simulink model "gm_Test_DOA"  (R2020b)
settings: Solver=ode4  StartTime=0.0  StopTime=0.16  RelTol=1e-3
undefined symbols (not defined in the file or in its folder): f_range, FFT_LENGTH, InvMp, Sampling_rate
libraries: dsphdlmathfun x4, dsphdlxfrm x4, hdlsllib x1
(part 1 of 2)
settings Model: Creator=tigro  LastModifiedBy=franc
settings OptimizationCC: BlockReduction=off  ConditionallyExecuteInputs=off  DefaultParameterBehavior=Inlined  OptimizeBlockIOStorage=off  EnhancedBackFolding=on  PassReuseOutputArgsAs=Individual arguments  OptimizeBlockOrder=speed  DifferentSizesBufferReuse=on  EfficientTunableParamExpr=on
settings DebuggingCC: AlgebraicLoopMsg=error  InheritedTsInSrcMsg=none  ParameterOverflowMsg=none  ParameterTunabilityLossMsg=error  AllowAutomaticUnitConversions=off
settings HardwareCC: ProdBitPerPointer=32  ProdBitPerSizeT=32  ProdBitPerPtrDiffT=32  ProdLargestAtomicFloat=None  ProdIntDivRoundTo=Undefined  ProdEndianess=Unspecified  ProdWordSize=32  ProdHWDeviceType=ASIC/FPGA->ASIC/FPGA  TargetBitPerPointer=64  TargetBitPerSizeT=64  TargetBitPerPtrDiffT=64  TargetLongLongMode=on  TargetIntDivRoundTo=Zero  TargetEndianess=LittleEndian  TargetWordSize=64  TargetHWDeviceType=Generic->Custom  ProdEqTarget=off
settings SFSimCC: MATLABDynamicMemAlloc=off
settings RTWCC: Description=SystemVerilog DPI Component Generator  SystemTargetFile=systemverilog_dpi_ert.tlc  TemplateMakefile=systemverilog_dpi_ert_default_tmf
settings CodeAppCC: ForceParamTrailComments=on  IgnoreCustomStorageClasses=off  MaxIdLength=256  OperatorAnnotations=on  SimulinkDataObjDesc=on  SFDataObjDesc=on  InsertBlockDesc=on
settings DPIERTTargetCC: TargetFcnLib=ansi_tfl_table_tmw.mat  GenFloatMathFcnCalls=NOT IN USE  TargetLangStandard=C89/C90 (ANSI)  CodeReplacementLibrary=None  UtilityFuncGeneration=Auto  MultiwordTypeDef=System defined  MultiwordLength=2048  DynamicStringBufferSize=256  GenerateFullHeader=on  InferredTypesCompatibility=off  GenerateSampleERTMain=off  GenerateTestInterfaces=off  ModelReferenceCompliant=on  ParMdlRefBuildCompliant=on  CompOptLevelCompliant=off  ConcurrentExecutionCompliant=off  IncludeMdlTerminateFcn=on  CombineOutputUpdateFcns=off  CombineSignalStateStructs=on  GroupInternalDataByFunction=off  SuppressErrorStatus=off  IncludeFileDelimiter=Auto  ERTCustomFileBanners=on  SupportAbsoluteTime=on  LogVarNameModifier=rt_  MatFileLogging=off  CodeInterfacePackaging=Reusable function  PurelyIntegerCode=off  SupportNonFinite=on  SupportComplex=on  SupportContinuousTime=on  SupportNonInlinedSFcns=on  RemoveDisableFunc=off  RemoveResetFunc=on  SupportVariableSizeSignals=off  ParenthesesLevel=Nominal  CastingMode=Nominal  MATLABClassNameForMDSCustomization=Simulink.SoftwareTarget.TargetSpecificTriggerConfigurationBase  ModelStepFunctionPrototypeControlCompliant=on  CPPClassGenCompliant=off  AutosarCompliant=off  MDXCompliant=off  GRTInterface=off  GenerateAllocFcn=on  UseToolchainInfoCompliant=on  GenerateSharedConstants=on  CoderGroups=[]  AccessMethods=[]  LookupTableObjectStructAxisOrder=1,2,3,4,...  LUTObjectStructOrderExplicitValues=Size,Breakpoints,Table  LUTObjectStructOrderEvenSpacing=Size,Breakpoints,Table  ArrayLayout=Column-major  UnsupportedSFcnMsg=error  ERTHeaderFileRootName=$R$E  ERTSourceFileRootName=$R$E  ERTDataFileRootName=$R_data  GenerateASAP2=off  DSAsUniqueAccess=off  ExtMode=off  ExtModeTransport=0  ExtModeStaticAlloc=off  ExtModeStaticAllocSize=1000000  ExtModeTesting=off  ExtModeMexFile=ext_comm  ExtModeIntrfLevel=Level1  InlinedParameterPlacement=NonHierarchical  TargetOS=BareBoardExample  MultiInstanceErrorCode=Error  RootIOFormat=Part of model data structure  RTWCAPISignals=on  RTWCAPIParams=off  RTWCAPIStates=off  RTWCAPIRootIO=off  ERTSrcFileBannerTemplate=ert_code_template.cgt  ERTHdrFileBannerTemplate=ert_code_template.cgt  ERTDataSrcFileTemplate=ert_code_template.cgt  ERTDataHdrFileTemplate=ert_code_template.cgt  ERTCustomFileTemplate=example_file_process.tlc  EnableDataOwnership=off  SignalDisplayLevel=10  ParamTuneLevel=10  GlobalDataDefinition=Auto  DataDefinitionFile=global.c  GlobalDataReference=Auto  ERTFilePackagingFormat=Modular  RateTransitionBlockCode=Inline  DataReferenceFile=global.h  PreserveExpressionOrder=off  PreserveIfCondition=off  ConvertIfToSwitch=on  PreserveExternInFcnDecls=on  PreserveStaticInFcnDecls=on  SuppressUnreachableDefaultCases=on  EnableSignedLeftShifts=on  EnableSignedRightShifts=on  IndentStyle=K&R  IndentSize=2  NewlineStyle=Default  MaxLineWidth=80  EnableUserReplacementTypes=off  MaxIdInt64=MAX_int64_T  MinIdInt64=MIN_int64_T  MaxIdUint64=MAX_uint64_T  MaxIdInt32=MAX_int32_T  MinIdInt32=MIN_int32_T  MaxIdUint32=MAX_uint32_T  MaxIdInt16=MAX_int16_T  MinIdInt16=MIN_int16_T  MaxIdUint16=MAX_uint16_T  MaxIdInt8=MAX_int8_T  MinIdInt8=MIN_int8_T  MaxIdUint8=MAX_uint8_T  BooleanTrueId=true  BooleanFalseId=false  MemSecPackage=--- None ---  MemSecDataConstants=Default  MemSecDataIO=Default  MemSecDataInternal=Default  MemSecDataParameters=Default  MemSecFuncInitTerm=Default  MemSecFuncExecute=Default  MemSecFuncSharedUtil=Default  GroupConstants=Default  GroupRootInputs=Default  GroupRootOutputs=Default  GroupInternal=Default  GroupParameters=Default  GroupDataTransfer=Default  GroupSharedLocalDataStores=Default  GroupInstanceSpecificParameters=Default  GroupModelData=Default  ArrayContainerType=C-style array  DPICustomizeSystemVerilogCode=off  DPISystemVerilogTemplate=svdpi_event.vgt  DPIReportRunTimeError=off  DPIRunTimeErrorSeverity=Fatal  DPIGenerateTestBench=off  DPITestBenchSimulator=Mentor Graphics Questasim  DPITestPointAccessFcnInterface=None  DPIFixedPointDataType=CompatibleCType  DPIPortConnection=Port list  DPICompositeDataType=Flattened

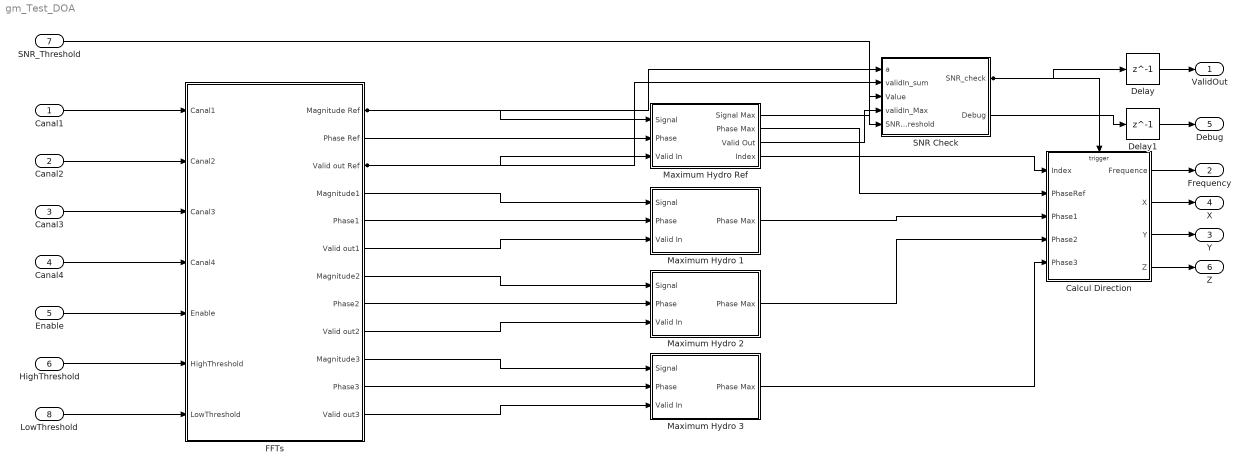
== system gm_Test_DOA ==
  Canal1 : Inport  OutDataTypeStr=uint16  PortDimensions=1  SampleTime=1e-07
  Canal2 : Inport  Port=2  OutDataTypeStr=uint16  PortDimensions=1  SampleTime=1e-07
  Canal3 : Inport  Port=3  OutDataTypeStr=uint16  PortDimensions=1  SampleTime=1e-07
  Canal4 : Inport  Port=4  OutDataTypeStr=uint16  PortDimensions=1  SampleTime=1e-07
  Enable : Inport  Port=5  OutDataTypeStr=boolean  PortDimensions=1  SampleTime=1e-07
  HighThreshold : Inport  Port=6  OutDataTypeStr=uint16  PortDimensions=1  SampleTime=1e-07
  SNR_Threshold : Inport  Port=7  OutDataTypeStr=uint8  PortDimensions=1  SampleTime=1e-07
  LowThreshold : Inport  Port=8  OutDataTypeStr=uint16  PortDimensions=1  SampleTime=1e-07
  Calcul Direction : Subsystem
  Delay : Delay  DelayLength=1
  Delay1 : Delay  DelayLength=1
  FFTs : Subsystem
  Maximum Hydro 1 : Subsystem
  Maximum Hydro 2 : Subsystem
  Maximum Hydro 3 : Subsystem
  Maximum Hydro Ref : Subsystem
  SNR Check : Subsystem
  ValidOut : Outport
  Frequency : Outport  Port=2
  Y : Outport  Port=3
  X : Outport  Port=4
  Debug : Outport  Port=5
  Z : Outport  Port=6
  wires:
  Canal1/1 -> FFTs/1(Canal1)
  Canal2/1 -> FFTs/2(Canal2)
  Canal3/1 -> FFTs/3(Canal3)
  Canal4/1 -> FFTs/4(Canal4)
  Enable/1 -> FFTs/5(Enable)
  HighThreshold/1 -> FFTs/6(HighThreshold)
  SNR_Threshold/1 -> SNR Check/5(SNR_Threshold)
  LowThreshold/1 -> FFTs/7(LowThreshold)
  Calcul Direction/1(Frequence) -> Frequency/1
  Calcul Direction/2(X) -> X/1
  Calcul Direction/3(Y) -> Y/1
  Calcul Direction/4(Z) -> Z/1
  Delay/1 -> ValidOut/1
  Delay1/1 -> Debug/1
  FFTs/1(Magnitude Ref) -> SNR Check/1(a), Maximum Hydro Ref/1(Signal)
  FFTs/2(Phase Ref) -> Maximum Hydro Ref/2(Phase)
  FFTs/3(Valid out Ref) -> SNR Check/2(validIn_sum), Maximum Hydro Ref/3(Valid In)
  FFTs/4(Magnitude1) -> Maximum Hydro 1/1(Signal)
  FFTs/5(Phase1) -> Maximum Hydro 1/2(Phase)
  FFTs/6(Valid out1) -> Maximum Hydro 1/3(Valid In)
  FFTs/7(Magnitude2) -> Maximum Hydro 2/1(Signal)
  FFTs/8(Phase2) -> Maximum Hydro 2/2(Phase)
  FFTs/9(Valid out2) -> Maximum Hydro 2/3(Valid In)
  FFTs/10(Magnitude3) -> Maximum Hydro 3/1(Signal)
  FFTs/11(Phase3) -> Maximum Hydro 3/2(Phase)
  FFTs/12(Valid out3) -> Maximum Hydro 3/3(Valid In)
  Maximum Hydro 1/1(Phase Max) -> Calcul Direction/3(Phase1)
  Maximum Hydro 2/1(Phase Max) -> Calcul Direction/4(Phase2)
  Maximum Hydro 3/1(Phase Max) -> Calcul Direction/5(Phase3)
  Maximum Hydro Ref/1(Signal Max) -> SNR Check/3(" Value")
  Maximum Hydro Ref/2(Phase Max) -> Calcul Direction/2(PhaseRef)
  Maximum Hydro Ref/3(Valid Out) -> SNR Check/4(validIn_Max)
  Maximum Hydro Ref/4(Index) -> Calcul Direction/1(Index)
  SNR Check/1(SNR_check) -> Delay/1, Calcul Direction/Trigger
  SNR Check/2(Debug) -> Delay1/1

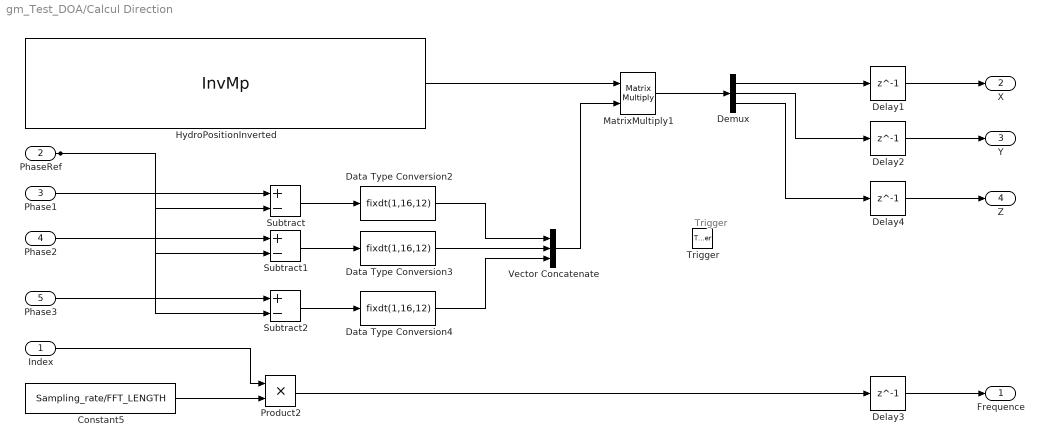
== system gm_Test_DOA/Calcul Direction ==
  note: Trigger
  Index : Inport  OutDataTypeStr=fixdt(0, 17, 0)  PortDimensions=1
  PhaseRef : Inport  Port=2  OutDataTypeStr=fixdt(1, 20, 17)  PortDimensions=1
  Phase1 : Inport  Port=3  OutDataTypeStr=fixdt(1, 20, 17)  PortDimensions=1
  Phase2 : Inport  Port=4  OutDataTypeStr=fixdt(1, 20, 17)  PortDimensions=1
  Phase3 : Inport  Port=5  OutDataTypeStr=fixdt(1, 20, 17)  PortDimensions=1
  Trigger : TriggerPort  VariantControl=(inherit)  PortDimensions=1  OutDataTypeStr=boolean
  Constant5 : Constant  Value=Sampling_rate/FFT_LENGTH  OutDataTypeStr=fixdt(0,10)  SampleTime=-1
  Data Type Conversion2 : DataTypeConversion  OutDataTypeStr=fixdt(1,16,12)
  Data Type Conversion3 : DataTypeConversion  OutDataTypeStr=fixdt(1,16,12)
  Data Type Conversion4 : DataTypeConversion  OutDataTypeStr=fixdt(1,16,12)
  Delay{1..4} (4 alike) : Delay  DelayLength=1
  Demux : Demux  Outputs=3
  HydroPositionInverted : Constant  Value=InvMp  VectorParams1D=off  OutDataTypeStr=fixdt(1,15,7)
  MatrixMultiply1 : Product  Multiplication=Matrix(*)
  Product2 : Product
  Subtract : Sum  Inputs=+-
  Subtract1 : Sum  Inputs=+-
  Subtract2 : Sum  Inputs=+-
  Vector Concatenate : Concatenate  NumInputs=3  Mode=Multidimensional array
  Frequence : Outport  InitialOutput=0
  X : Outport  Port=2  InitialOutput=0
  Y : Outport  Port=3  InitialOutput=0
  Z : Outport  Port=4  InitialOutput=0
  wires:
  Index/1 -> Product2/1
  PhaseRef/1 -> Subtract2/2, Subtract1/2, Subtract/2
  Phase1/1 -> Subtract/1
  Phase2/1 -> Subtract1/1
  Phase3/1 -> Subtract2/1
  Constant5/1 -> Product2/2
  Data Type Conversion2/1 -> Vector Concatenate/1
  Data Type Conversion3/1 -> Vector Concatenate/2
  Data Type Conversion4/1 -> Vector Concatenate/3
  Delay1/1 -> X/1
  Delay2/1 -> Y/1
  Delay3/1 -> Frequence/1
  Delay4/1 -> Z/1
  Demux/1 -> Delay1/1
  Demux/2 -> Delay2/1
  Demux/3 -> Delay4/1
  HydroPositionInverted/1 -> MatrixMultiply1/1
  MatrixMultiply1/1 -> Demux/1
  Product2/1 -> Delay3/1
  Subtract/1 -> Data Type Conversion2/1
  Subtract1/1 -> Data Type Conversion3/1
  Subtract2/1 -> Data Type Conversion4/1
  Vector Concatenate/1 -> MatrixMultiply1/2

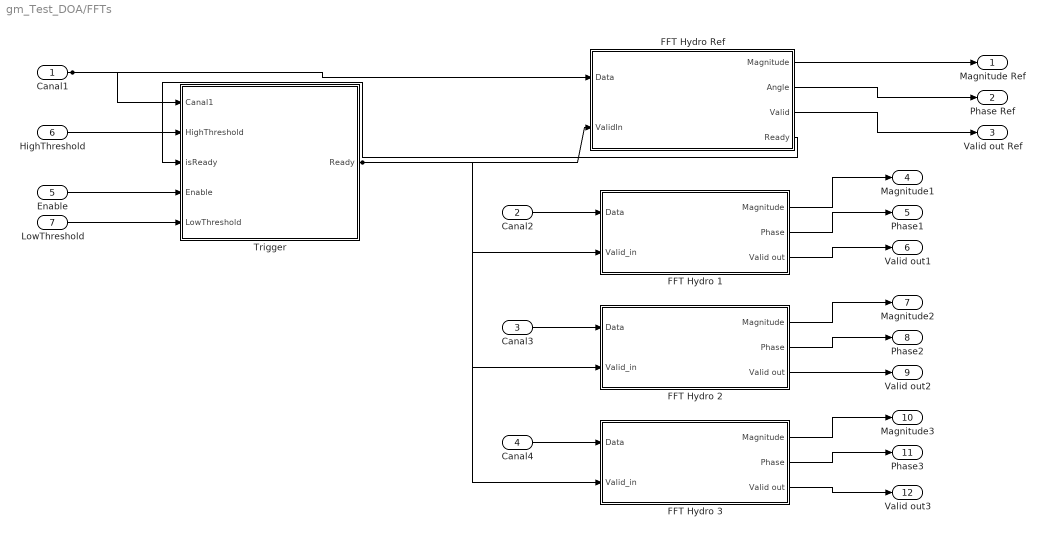
== system gm_Test_DOA/FFTs ==
  Canal1 : Inport  OutDataTypeStr=uint16  PortDimensions=1  SampleTime=1e-07
  Canal2 : Inport  Port=2  OutDataTypeStr=uint16  PortDimensions=1  SampleTime=1e-07
  Canal3 : Inport  Port=3  OutDataTypeStr=uint16  PortDimensions=1  SampleTime=1e-07
  Canal4 : Inport  Port=4  OutDataTypeStr=uint16  PortDimensions=1  SampleTime=1e-07
  Enable : Inport  Port=5  OutDataTypeStr=boolean  PortDimensions=1  SampleTime=1e-07
  HighThreshold : Inport  Port=6  OutDataTypeStr=uint16  PortDimensions=1  SampleTime=1e-07
  LowThreshold : Inport  Port=7  OutDataTypeStr=uint16  PortDimensions=1  SampleTime=1e-07
  FFT Hydro 1 : Subsystem
  FFT Hydro 2 : Subsystem
  FFT Hydro 3 : Subsystem
  FFT Hydro Ref : Subsystem
  Trigger : Subsystem
  Magnitude Ref : Outport
  Phase Ref : Outport  Port=2
  Valid out Ref : Outport  Port=3
  Magnitude1 : Outport  Port=4
  Phase1 : Outport  Port=5
  Valid out1 : Outport  Port=6
  Magnitude2 : Outport  Port=7
  Phase2 : Outport  Port=8
  Valid out2 : Outport  Port=9
  Magnitude3 : Outport  Port=10
  Phase3 : Outport  Port=11
  Valid out3 : Outport  Port=12
  wires:
  Canal1/1 -> FFT Hydro Ref/1(Data), Trigger/1(Canal1)
  Canal2/1 -> FFT Hydro 1/1(Data)
  Canal3/1 -> FFT Hydro 2/1(Data)
  Canal4/1 -> FFT Hydro 3/1(Data)
  Enable/1 -> Trigger/4(Enable)
  HighThreshold/1 -> Trigger/2(HighThreshold)
  LowThreshold/1 -> Trigger/5(LowThreshold)
  FFT Hydro 1/1(Magnitude) -> Magnitude1/1
  FFT Hydro 1/2(Phase) -> Phase1/1
  FFT Hydro 1/3(Valid out) -> Valid out1/1
  FFT Hydro 2/1(Magnitude) -> Magnitude2/1
  FFT Hydro 2/2(Phase) -> Phase2/1
  FFT Hydro 2/3(Valid out) -> Valid out2/1
  FFT Hydro 3/1(Magnitude) -> Magnitude3/1
  FFT Hydro 3/2(Phase) -> Phase3/1
  FFT Hydro 3/3(Valid out) -> Valid out3/1
  FFT Hydro Ref/1(Magnitude) -> Magnitude Ref/1
  FFT Hydro Ref/2(Angle) -> Phase Ref/1
  FFT Hydro Ref/3(Valid) -> Valid out Ref/1
  FFT Hydro Ref/4(Ready) -> Trigger/3(isReady)
  Trigger/1(Ready) -> FFT Hydro Ref/2(ValidIn), FFT Hydro 3/2(Valid_in), FFT Hydro 2/2(Valid_in), FFT Hydro 1/2(Valid_in)

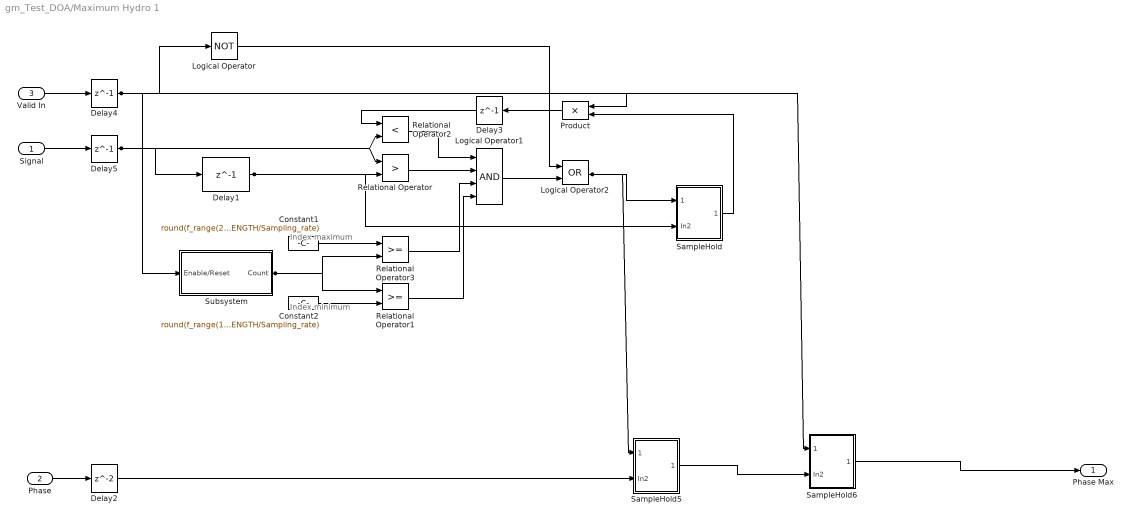
== system gm_Test_DOA/Maximum Hydro 1 ==
  note: Index maximum
  note: Index minimum
  Signal : Inport  OutDataTypeStr=fixdt(1, 18, 0)  PortDimensions=1  SampleTime=1e-07
  Phase : Inport  Port=2  OutDataTypeStr=fixdt(1, 20, 17)  PortDimensions=1  SampleTime=1e-07
  Valid In : Inport  Port=3  OutDataTypeStr=boolean  PortDimensions=1  SampleTime=1e-07
  Constant1 : Constant  Value=round(f_range(2)*FFT_LENGTH/Sampling_rate)  OutDataTypeStr=fixdt(0,6)  SampleTime=-1
  Constant2 : Constant  Value=round(f_range(1)*FFT_LENGTH/Sampling_rate)  OutDataTypeStr=fixdt(0,6)  SampleTime=-1
  Delay{1,3..5} (4 alike) : Delay  DelayLength=1  InitialCondition=0  UseCircularBuffer=on
  Delay2 : Delay  InitialCondition=0  UseCircularBuffer=on
  Logical Operator : Logic  Operator=NOT  IconShape=distinctive  AllPortsSameDT=off  OutDataTypeStr=boolean
  Logical Operator1 : Logic  Inputs=4  AllPortsSameDT=off  OutDataTypeStr=boolean
  Logical Operator2 : Logic  Operator=OR  AllPortsSameDT=off  OutDataTypeStr=boolean
  Product : Product
  Relational Operator : RelationalOperator  Operator=>  OutDataTypeStr=boolean  RndMeth=Nearest
  Relational Operator1 : RelationalOperator  OutDataTypeStr=boolean  RndMeth=Nearest
  Relational Operator2 : RelationalOperator  Operator=<  OutDataTypeStr=boolean  RndMeth=Nearest
  Relational Operator3 : RelationalOperator  OutDataTypeStr=boolean  RndMeth=Nearest
  SampleHold : Subsystem
  SampleHold5 : Subsystem
  SampleHold6 : Subsystem
  Subsystem : Subsystem
  Phase Max : Outport  VectorParamsAs1DForOutWhenUnconnected=off
  wires:
  Signal/1 -> Delay5/1
  Phase/1 -> Delay2/1
  Valid In/1 -> Delay4/1
  Constant1/1 -> Relational Operator3/1
  Constant2/1 -> Relational Operator1/2
  Delay1/1 -> Relational Operator/2, SampleHold/2(In2)
  Delay2/1 -> SampleHold5/2(In2)
  Delay3/1 -> Relational Operator2/1
  Delay4/1 -> Product/1, Logical Operator/1, SampleHold6/1(Trigger), Subsystem/1(Enable/Reset)
  Delay5/1 -> Relational Operator2/2, Relational Operator/1, Delay1/1
  Logical Operator/1 -> Logical Operator2/1
  Logical Operator1/1 -> Logical Operator2/2
  Logical Operator2/1 -> SampleHold5/1(Trigger), SampleHold/1(Trigger)
  Product/1 -> Delay3/1
  Relational Operator/1 -> Logical Operator1/2
  Relational Operator1/1 -> Logical Operator1/4
  Relational Operator2/1 -> Logical Operator1/1
  Relational Operator3/1 -> Logical Operator1/3
  SampleHold/1(" ") -> Product/2
  SampleHold5/1(" ") -> SampleHold6/2(In2)
  SampleHold6/1(" ") -> Phase Max/1
  Subsystem/1(Count) -> Relational Operator3/2, Relational Operator1/1

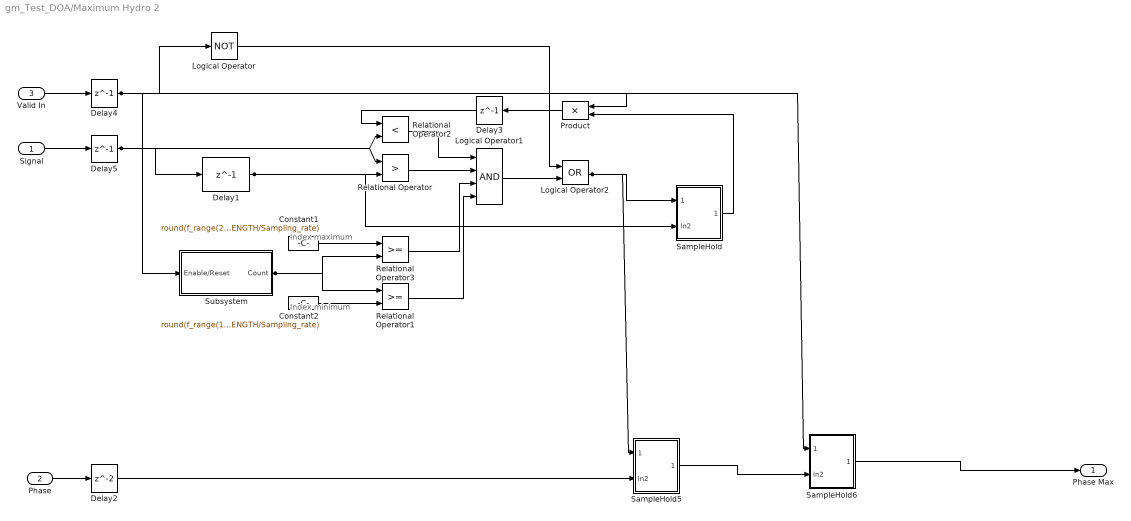
== system gm_Test_DOA/Maximum Hydro 2 ==
  note: Index maximum
  note: Index minimum
  Signal : Inport  OutDataTypeStr=fixdt(1, 18, 0)  PortDimensions=1  SampleTime=1e-07
  Phase : Inport  Port=2  OutDataTypeStr=fixdt(1, 20, 17)  PortDimensions=1  SampleTime=1e-07
  Valid In : Inport  Port=3  OutDataTypeStr=boolean  PortDimensions=1  SampleTime=1e-07
  Constant1 : Constant  Value=round(f_range(2)*FFT_LENGTH/Sampling_rate)  OutDataTypeStr=fixdt(0,6)  SampleTime=-1
  Constant2 : Constant  Value=round(f_range(1)*FFT_LENGTH/Sampling_rate)  OutDataTypeStr=fixdt(0,6)  SampleTime=-1
  Delay{1,3..5} (4 alike) : Delay  DelayLength=1  InitialCondition=0  UseCircularBuffer=on
  Delay2 : Delay  InitialCondition=0  UseCircularBuffer=on
  Logical Operator : Logic  Operator=NOT  IconShape=distinctive  AllPortsSameDT=off  OutDataTypeStr=boolean
  Logical Operator1 : Logic  Inputs=4  AllPortsSameDT=off  OutDataTypeStr=boolean
  Logical Operator2 : Logic  Operator=OR  AllPortsSameDT=off  OutDataTypeStr=boolean
  Product : Product
  Relational Operator : RelationalOperator  Operator=>  OutDataTypeStr=boolean  RndMeth=Nearest
  Relational Operator1 : RelationalOperator  OutDataTypeStr=boolean  RndMeth=Nearest
  Relational Operator2 : RelationalOperator  Operator=<  OutDataTypeStr=boolean  RndMeth=Nearest
  Relational Operator3 : RelationalOperator  OutDataTypeStr=boolean  RndMeth=Nearest
  SampleHold : Subsystem
  SampleHold5 : Subsystem
  SampleHold6 : Subsystem
  Subsystem : Subsystem
  Phase Max : Outport  VectorParamsAs1DForOutWhenUnconnected=off
  wires:
  Signal/1 -> Delay5/1
  Phase/1 -> Delay2/1
  Valid In/1 -> Delay4/1
  Constant1/1 -> Relational Operator3/1
  Constant2/1 -> Relational Operator1/2
  Delay1/1 -> Relational Operator/2, SampleHold/2(In2)
  Delay2/1 -> SampleHold5/2(In2)
  Delay3/1 -> Relational Operator2/1
  Delay4/1 -> Product/1, Logical Operator/1, SampleHold6/1(Trigger), Subsystem/1(Enable/Reset)
  Delay5/1 -> Relational Operator2/2, Relational Operator/1, Delay1/1
  Logical Operator/1 -> Logical Operator2/1
  Logical Operator1/1 -> Logical Operator2/2
  Logical Operator2/1 -> SampleHold5/1(Trigger), SampleHold/1(Trigger)
  Product/1 -> Delay3/1
  Relational Operator/1 -> Logical Operator1/2
  Relational Operator1/1 -> Logical Operator1/4
  Relational Operator2/1 -> Logical Operator1/1
  Relational Operator3/1 -> Logical Operator1/3
  SampleHold/1(" ") -> Product/2
  SampleHold5/1(" ") -> SampleHold6/2(In2)
  SampleHold6/1(" ") -> Phase Max/1
  Subsystem/1(Count) -> Relational Operator3/2, Relational Operator1/1

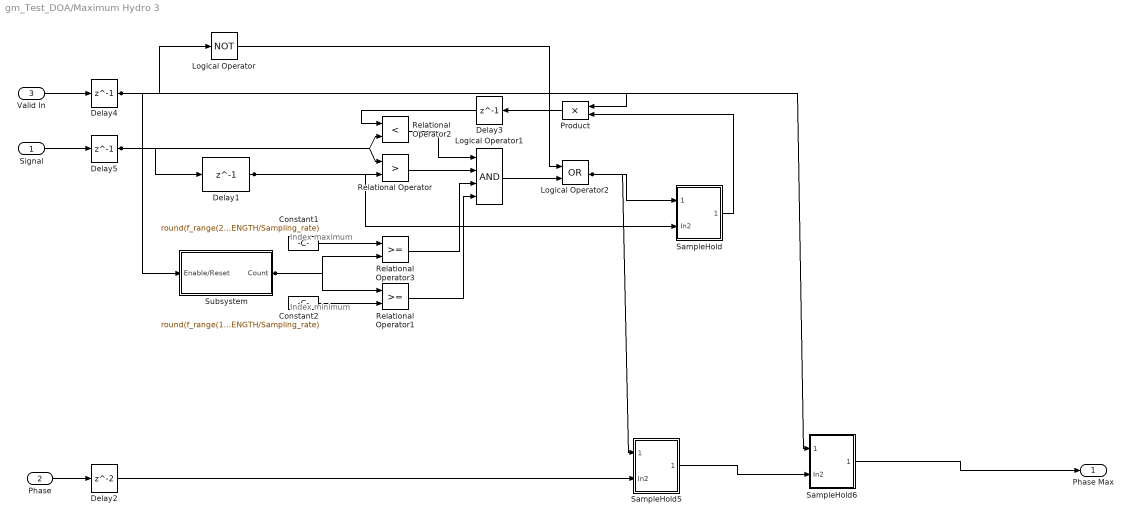
== system gm_Test_DOA/Maximum Hydro 3 ==
  note: Index maximum
  note: Index minimum
  Signal : Inport  OutDataTypeStr=fixdt(1, 18, 0)  PortDimensions=1  SampleTime=1e-07
  Phase : Inport  Port=2  OutDataTypeStr=fixdt(1, 20, 17)  PortDimensions=1  SampleTime=1e-07
  Valid In : Inport  Port=3  OutDataTypeStr=boolean  PortDimensions=1  SampleTime=1e-07
  Constant1 : Constant  Value=round(f_range(2)*FFT_LENGTH/Sampling_rate)  OutDataTypeStr=fixdt(0,6)  SampleTime=-1
  Constant2 : Constant  Value=round(f_range(1)*FFT_LENGTH/Sampling_rate)  OutDataTypeStr=fixdt(0,6)  SampleTime=-1
  Delay{1,3..5} (4 alike) : Delay  DelayLength=1  InitialCondition=0  UseCircularBuffer=on
  Delay2 : Delay  InitialCondition=0  UseCircularBuffer=on
  Logical Operator : Logic  Operator=NOT  IconShape=distinctive  AllPortsSameDT=off  OutDataTypeStr=boolean
  Logical Operator1 : Logic  Inputs=4  AllPortsSameDT=off  OutDataTypeStr=boolean
  Logical Operator2 : Logic  Operator=OR  AllPortsSameDT=off  OutDataTypeStr=boolean
  Product : Product
  Relational Operator : RelationalOperator  Operator=>  OutDataTypeStr=boolean  RndMeth=Nearest
  Relational Operator1 : RelationalOperator  OutDataTypeStr=boolean  RndMeth=Nearest
  Relational Operator2 : RelationalOperator  Operator=<  OutDataTypeStr=boolean  RndMeth=Nearest
  Relational Operator3 : RelationalOperator  OutDataTypeStr=boolean  RndMeth=Nearest
  SampleHold : Subsystem
  SampleHold5 : Subsystem
  SampleHold6 : Subsystem
  Subsystem : Subsystem
  Phase Max : Outport  VectorParamsAs1DForOutWhenUnconnected=off
  wires:
  Signal/1 -> Delay5/1
  Phase/1 -> Delay2/1
  Valid In/1 -> Delay4/1
  Constant1/1 -> Relational Operator3/1
  Constant2/1 -> Relational Operator1/2
  Delay1/1 -> Relational Operator/2, SampleHold/2(In2)
  Delay2/1 -> SampleHold5/2(In2)
  Delay3/1 -> Relational Operator2/1
  Delay4/1 -> Product/1, Logical Operator/1, SampleHold6/1(Trigger), Subsystem/1(Enable/Reset)
  Delay5/1 -> Relational Operator2/2, Relational Operator/1, Delay1/1
  Logical Operator/1 -> Logical Operator2/1
  Logical Operator1/1 -> Logical Operator2/2
  Logical Operator2/1 -> SampleHold5/1(Trigger), SampleHold/1(Trigger)
  Product/1 -> Delay3/1
  Relational Operator/1 -> Logical Operator1/2
  Relational Operator1/1 -> Logical Operator1/4
  Relational Operator2/1 -> Logical Operator1/1
  Relational Operator3/1 -> Logical Operator1/3
  SampleHold/1(" ") -> Product/2
  SampleHold5/1(" ") -> SampleHold6/2(In2)
  SampleHold6/1(" ") -> Phase Max/1
  Subsystem/1(Count) -> Relational Operator3/2, Relational Operator1/1

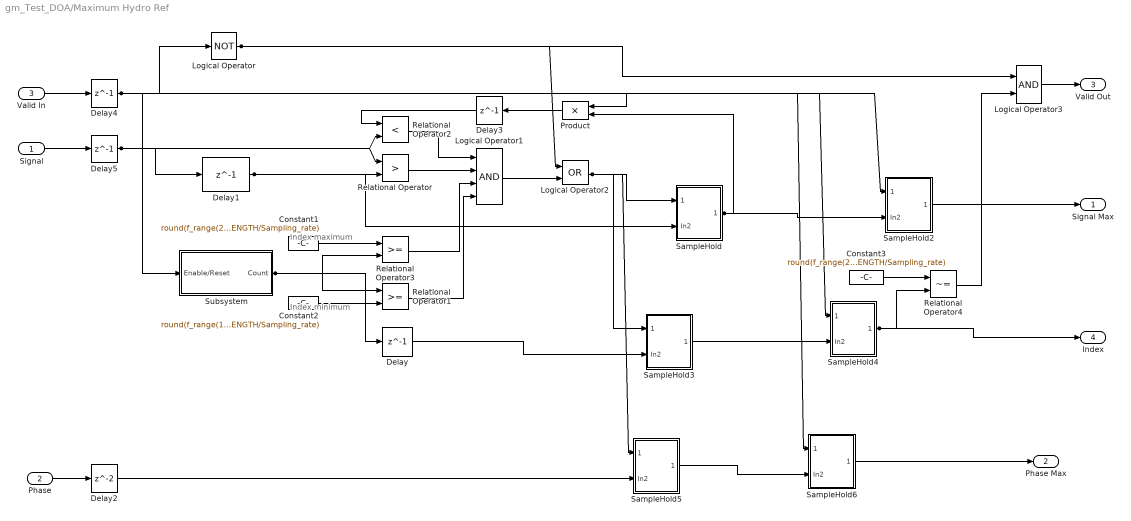
== system gm_Test_DOA/Maximum Hydro Ref ==
  note: Index maximum
  note: Index minimum
  Signal : Inport  OutDataTypeStr=fixdt(1, 18, 0)  PortDimensions=1  SampleTime=1e-07
  Phase : Inport  Port=2  OutDataTypeStr=fixdt(1, 20, 17)  PortDimensions=1  SampleTime=1e-07
  Valid In : Inport  Port=3  OutDataTypeStr=boolean  PortDimensions=1  SampleTime=1e-07
  Constant1 : Constant  Value=round(f_range(2)*FFT_LENGTH/Sampling_rate)  OutDataTypeStr=fixdt(0,6)  SampleTime=-1
  Constant2 : Constant  Value=round(f_range(1)*FFT_LENGTH/Sampling_rate)  OutDataTypeStr=fixdt(0,6)  SampleTime=-1
  Constant3 : Constant  Value=round(f_range(2)*FFT_LENGTH/Sampling_rate)  OutDataTypeStr=fixdt(0,6)  SampleTime=-1
  Delay : Delay  DelayLength=1  InitialCondition=0
  Delay{1,3..5} (4 alike) : Delay  DelayLength=1  InitialCondition=0  UseCircularBuffer=on
  Delay2 : Delay  InitialCondition=0  UseCircularBuffer=on
  Logical Operator : Logic  Operator=NOT  IconShape=distinctive  AllPortsSameDT=off  OutDataTypeStr=boolean
  Logical Operator1 : Logic  Inputs=4  AllPortsSameDT=off  OutDataTypeStr=boolean
  Logical Operator2 : Logic  Operator=OR  AllPortsSameDT=off  OutDataTypeStr=boolean
  Logical Operator3 : Logic  AllPortsSameDT=off  OutDataTypeStr=boolean
  Product : Product
  Relational Operator : RelationalOperator  Operator=>  OutDataTypeStr=boolean  RndMeth=Nearest
  Relational Operator1 : RelationalOperator  OutDataTypeStr=boolean  RndMeth=Nearest
  Relational Operator2 : RelationalOperator  Operator=<  OutDataTypeStr=boolean  RndMeth=Nearest
  Relational Operator3 : RelationalOperator  OutDataTypeStr=boolean  RndMeth=Nearest
  Relational Operator4 : RelationalOperator  Operator=~=  OutDataTypeStr=boolean  RndMeth=Nearest
  SampleHold : Subsystem
  SampleHold2 : Subsystem
  SampleHold3 : Subsystem
  SampleHold4 : Subsystem
  SampleHold5 : Subsystem
  SampleHold6 : Subsystem
  Subsystem : Subsystem
  Signal Max : Outport  VectorParamsAs1DForOutWhenUnconnected=off
  Phase Max : Outport  Port=2  VectorParamsAs1DForOutWhenUnconnected=off
  Valid Out : Outport  Port=3  VectorParamsAs1DForOutWhenUnconnected=off
  Index : Outport  Port=4  VectorParamsAs1DForOutWhenUnconnected=off
  wires:
  Signal/1 -> Delay5/1
  Phase/1 -> Delay2/1
  Valid In/1 -> Delay4/1
  Constant1/1 -> Relational Operator3/1
  Constant2/1 -> Relational Operator1/2
  Constant3/1 -> Relational Operator4/1
  Delay/1 -> SampleHold3/2(In2)
  Delay1/1 -> Relational Operator/2, SampleHold/2(In2)
  Delay2/1 -> SampleHold5/2(In2)
  Delay3/1 -> Relational Operator2/1
  Delay4/1 -> Product/1, Logical Operator/1, SampleHold6/1(Trigger), SampleHold4/1(Trigger), SampleHold2/1(Trigger), Subsystem/1(Enable/Reset)
  Delay5/1 -> Relational Operator2/2, Relational Operator/1, Delay1/1
  Logical Operator/1 -> Logical Operator3/1, Logical Operator2/1
  Logical Operator1/1 -> Logical Operator2/2
  Logical Operator2/1 -> SampleHold5/1(Trigger), SampleHold3/1(Trigger), SampleHold/1(Trigger)
  Logical Operator3/1 -> Valid Out/1
  Product/1 -> Delay3/1
  Relational Operator/1 -> Logical Operator1/2
  Relational Operator1/1 -> Logical Operator1/4
  Relational Operator2/1 -> Logical Operator1/1
  Relational Operator3/1 -> Logical Operator1/3
  Relational Operator4/1 -> Logical Operator3/2
  SampleHold/1(" ") -> Product/2, SampleHold2/2(In2)
  SampleHold2/1(" ") -> Signal Max/1
  SampleHold3/1(" ") -> SampleHold4/2(In2)
  SampleHold4/1(" ") -> Relational Operator4/2, Index/1
  SampleHold5/1(" ") -> SampleHold6/2(In2)
  SampleHold6/1(" ") -> Phase Max/1
  Subsystem/1(Count) -> Relational Operator3/2, Relational Operator1/1, Delay/1

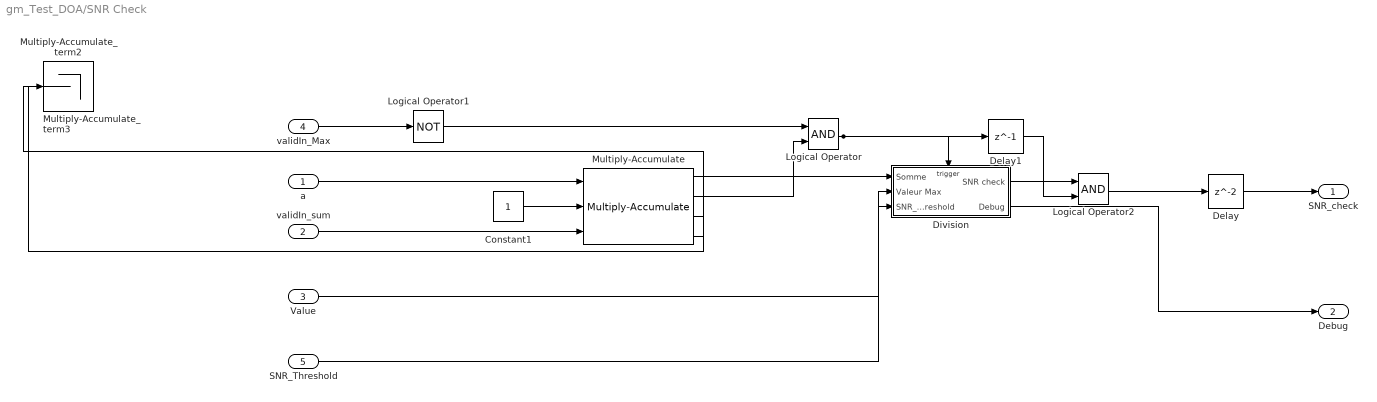
== system gm_Test_DOA/SNR Check ==
  a : Inport  OutDataTypeStr=fixdt(1, 18, 0)  PortDimensions=1  SampleTime=1e-07
  validIn_sum : Inport  Port=2  OutDataTypeStr=boolean  PortDimensions=1  SampleTime=1e-07
  " Value" : Inport  Port=3  OutDataTypeStr=fixdt(1, 18, 0)  PortDimensions=1  SampleTime=1e-07
  validIn_Max : Inport  Port=4  OutDataTypeStr=boolean  PortDimensions=1  SampleTime=1e-07
  SNR_Threshold : Inport  Port=5  OutDataTypeStr=uint8  PortDimensions=1  SampleTime=1e-07
  Constant1 : Constant  OutDataTypeStr=fixdt(1,18,0)  SampleTime=-1
  Delay : Delay
  Delay1 : Delay  DelayLength=1
  Division : Subsystem
  Logical Operator : Logic  AllPortsSameDT=off  OutDataTypeStr=boolean
  Logical Operator1 : Logic  Operator=NOT  AllPortsSameDT=off  OutDataTypeStr=boolean
  Logical Operator2 : Logic  AllPortsSameDT=off  OutDataTypeStr=boolean
  Multiply-Accumulate : hdlsllib/HDL Operations/Multiply-Accumulate  opMode=Streaming - using Number of Samples  initValueSetting=Dialog  initValue=0  initValueSetting2=Dialog  initValue2=0  initValueSetting3=Dialog  initValue3=0  num_samples=256  RndMeth2=Floor  RndMeth3=Floor  datatype2=Inherit: Inherit via back propagation  datatype3=fixdt(1,27,8)  validOut=on  endInandOut=on  startOut=on  countOut=on  dim=-1  DoSatur=off  parallel=off
      settings: SourceProductBaseCode=SL
  Multiply-Accumulate_term2 : Terminator
  Multiply-Accumulate_term3 : Terminator
  SNR_check : Outport
  Debug : Outport  Port=2
  wires:
  a/1 -> Multiply-Accumulate/1
  validIn_sum/1 -> Multiply-Accumulate/3
  " Value"/1 -> Division/2(" Valeur Max")
  validIn_Max/1 -> Logical Operator1/1
  SNR_Threshold/1 -> Division/3(SNR_Threshold)
  Constant1/1 -> Multiply-Accumulate/2
  Delay/1 -> SNR_check/1
  Delay1/1 -> Logical Operator2/2
  Division/1(SNR check) -> Logical Operator2/1
  Division/2(Debug) -> Debug/1
  Logical Operator/1 -> Delay1/1, Division/Trigger
  Logical Operator1/1 -> Logical Operator/1
  Logical Operator2/1 -> Delay/1
  Multiply-Accumulate/1 -> Division/1(Somme)
  Multiply-Accumulate/2 -> Logical Operator/2
  Multiply-Accumulate/3 -> Multiply-Accumulate_term2/1
  Multiply-Accumulate/4 -> Multiply-Accumulate_term3/1

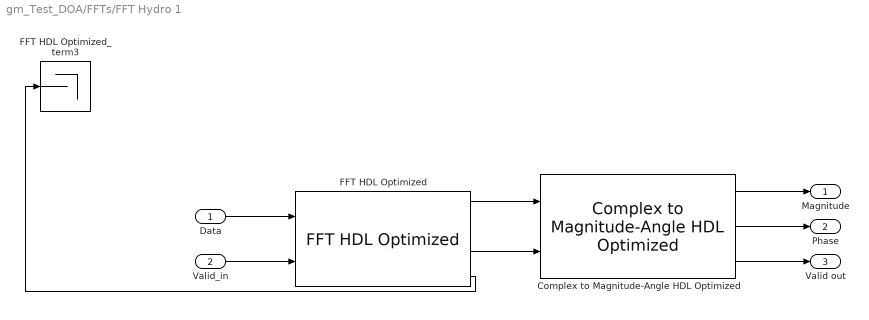
== system gm_Test_DOA/FFTs/FFT Hydro 1 ==
  Data : Inport  OutDataTypeStr=uint16  PortDimensions=1  SampleTime=1e-07
  Valid_in : Inport  Port=2  OutDataTypeStr=boolean  PortDimensions=1  SampleTime=1e-07
  Complex to Magnitude-Angle HDL Optimized : dsphdlmathfun/Complex to Magnitude-Angle HDL Optimized  NumIterationsSource=Property  NumIterations=CORDIC_Estimation  OutputFormat=Magnitude and angle  AngleFormat=Radians  ScaleOutput=on  SimulateUsing=Code generation
      settings: SourceProductBaseCode=DS
  FFT HDL Optimized : dsphdlxfrm/FFT HDL Optimized  FFTLength=FFT_LENGTH  Architecture=Burst Radix 2  ComplexMultiplication=Use 3 multipliers and 5 adders  BitReversedOutput=off  BitReversedInput=off  Normalize=on  SimulateUsing=Code generation  RoundingMethod=Floor  ResetInputPort=off  StartOutputPort=off  EndOutputPort=on
      settings: SourceProductBaseCode=DS
  FFT HDL Optimized_term3 : Terminator
  Magnitude : Outport
  Phase : Outport  Port=2
  Valid out : Outport  Port=3
  wires:
  Data/1 -> FFT HDL Optimized/1
  Valid_in/1 -> FFT HDL Optimized/2
  Complex to Magnitude-Angle HDL Optimized/1 -> Magnitude/1
  Complex to Magnitude-Angle HDL Optimized/2 -> Phase/1
  Complex to Magnitude-Angle HDL Optimized/3 -> Valid out/1
  FFT HDL Optimized/1 -> Complex to Magnitude-Angle HDL Optimized/1
  FFT HDL Optimized/3 -> Complex to Magnitude-Angle HDL Optimized/2
  FFT HDL Optimized/4 -> FFT HDL Optimized_term3/1

== system gm_Test_DOA/FFTs/FFT Hydro 2 ==
  Data : Inport  OutDataTypeStr=uint16  PortDimensions=1  SampleTime=1e-07
  Valid_in : Inport  Port=2  OutDataTypeStr=boolean  PortDimensions=1  SampleTime=1e-07
  Complex to Magnitude-Angle HDL Optimized : dsphdlmathfun/Complex to Magnitude-Angle HDL Optimized  NumIterationsSource=Property  NumIterations=CORDIC_Estimation  OutputFormat=Magnitude and angle  AngleFormat=Radians  ScaleOutput=on  SimulateUsing=Code generation
      settings: SourceProductBaseCode=DS
  FFT HDL Optimized : dsphdlxfrm/FFT HDL Optimized  FFTLength=FFT_LENGTH  Architecture=Burst Radix 2  ComplexMultiplication=Use 3 multipliers and 5 adders  BitReversedOutput=off  BitReversedInput=off  Normalize=on  SimulateUsing=Code generation  RoundingMethod=Floor  ResetInputPort=off  StartOutputPort=off  EndOutputPort=off
      settings: SourceProductBaseCode=DS
  Magnitude : Outport
  Phase : Outport  Port=2
  Valid out : Outport  Port=3
  wires:
  Data/1 -> FFT HDL Optimized/1
  Valid_in/1 -> FFT HDL Optimized/2
  Complex to Magnitude-Angle HDL Optimized/1 -> Magnitude/1
  Complex to Magnitude-Angle HDL Optimized/2 -> Phase/1
  Complex to Magnitude-Angle HDL Optimized/3 -> Valid out/1
  FFT HDL Optimized/1 -> Complex to Magnitude-Angle HDL Optimized/1
  FFT HDL Optimized/2 -> Complex to Magnitude-Angle HDL Optimized/2

== system gm_Test_DOA/FFTs/FFT Hydro 3 ==
  Data : Inport  OutDataTypeStr=uint16  PortDimensions=1  SampleTime=1e-07
  Valid_in : Inport  Port=2  OutDataTypeStr=boolean  PortDimensions=1  SampleTime=1e-07
  Complex to Magnitude-Angle HDL Optimized : dsphdlmathfun/Complex to Magnitude-Angle HDL Optimized  NumIterationsSource=Property  NumIterations=CORDIC_Estimation  OutputFormat=Magnitude and angle  AngleFormat=Radians  ScaleOutput=on  SimulateUsing=Code generation
      settings: SourceProductBaseCode=DS
  FFT HDL Optimized : dsphdlxfrm/FFT HDL Optimized  FFTLength=FFT_LENGTH  Architecture=Burst Radix 2  ComplexMultiplication=Use 3 multipliers and 5 adders  BitReversedOutput=off  BitReversedInput=off  Normalize=on  SimulateUsing=Code generation  RoundingMethod=Floor  ResetInputPort=off  StartOutputPort=off  EndOutputPort=off
      settings: SourceProductBaseCode=DS
  Magnitude : Outport
  Phase : Outport  Port=2
  Valid out : Outport  Port=3
  wires:
  Data/1 -> FFT HDL Optimized/1
  Valid_in/1 -> FFT HDL Optimized/2
  Complex to Magnitude-Angle HDL Optimized/1 -> Magnitude/1
  Complex to Magnitude-Angle HDL Optimized/2 -> Phase/1
  Complex to Magnitude-Angle HDL Optimized/3 -> Valid out/1
  FFT HDL Optimized/1 -> Complex to Magnitude-Angle HDL Optimized/1
  FFT HDL Optimized/2 -> Complex to Magnitude-Angle HDL Optimized/2

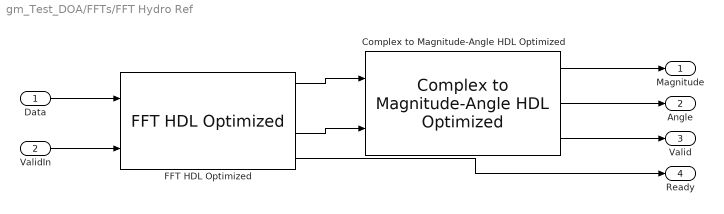
== system gm_Test_DOA/FFTs/FFT Hydro Ref ==
  Data : Inport  OutDataTypeStr=uint16  PortDimensions=1  SampleTime=1e-07
  ValidIn : Inport  Port=2  OutDataTypeStr=boolean  PortDimensions=1  SampleTime=1e-07
  Complex to Magnitude-Angle HDL Optimized : dsphdlmathfun/Complex to Magnitude-Angle HDL Optimized  NumIterationsSource=Property  NumIterations=CORDIC_Estimation  OutputFormat=Magnitude and angle  AngleFormat=Radians  ScaleOutput=on  SimulateUsing=Code generation
      settings: SourceProductBaseCode=DS
  FFT HDL Optimized : dsphdlxfrm/FFT HDL Optimized  FFTLength=FFT_LENGTH  Architecture=Burst Radix 2  ComplexMultiplication=Use 3 multipliers and 5 adders  BitReversedOutput=off  BitReversedInput=off  Normalize=on  SimulateUsing=Code generation  RoundingMethod=Floor  ResetInputPort=off  StartOutputPort=off  EndOutputPort=on
      settings: SourceProductBaseCode=DS
  Magnitude : Outport
  Angle : Outport  Port=2
  Valid : Outport  Port=3
  Ready : Outport  Port=4
  wires:
  Data/1 -> FFT HDL Optimized/1
  ValidIn/1 -> FFT HDL Optimized/2
  Complex to Magnitude-Angle HDL Optimized/1 -> Magnitude/1
  Complex to Magnitude-Angle HDL Optimized/2 -> Angle/1
  Complex to Magnitude-Angle HDL Optimized/3 -> Valid/1
  FFT HDL Optimized/1 -> Complex to Magnitude-Angle HDL Optimized/1
  FFT HDL Optimized/3 -> Complex to Magnitude-Angle HDL Optimized/2
  FFT HDL Optimized/4 -> Ready/1

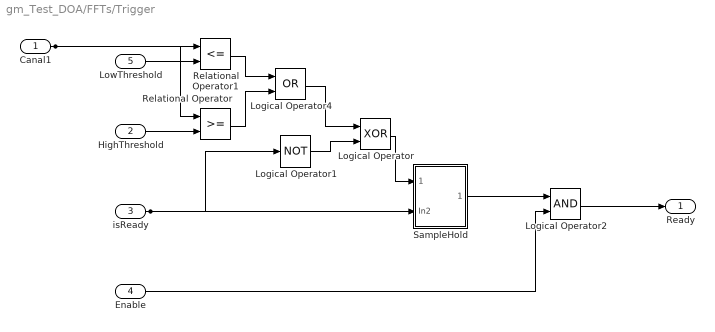
== system gm_Test_DOA/FFTs/Trigger ==
  Canal1 : Inport  OutDataTypeStr=uint16  PortDimensions=1  SampleTime=1e-07
  HighThreshold : Inport  Port=2  OutDataTypeStr=uint16  PortDimensions=1  SampleTime=1e-07
  isReady : Inport  Port=3  OutDataTypeStr=boolean  PortDimensions=1  SampleTime=1e-07
  Enable : Inport  Port=4  OutDataTypeStr=boolean  PortDimensions=1  SampleTime=1e-07
  LowThreshold : Inport  Port=5  OutDataTypeStr=uint16  PortDimensions=1  SampleTime=1e-07
  Logical Operator : Logic  Operator=XOR  AllPortsSameDT=off  OutDataTypeStr=boolean
  Logical Operator1 : Logic  Operator=NOT  IconShape=distinctive  AllPortsSameDT=off  OutDataTypeStr=boolean
  Logical Operator2 : Logic  AllPortsSameDT=off  OutDataTypeStr=boolean
  Logical Operator4 : Logic  Operator=OR  AllPortsSameDT=off  OutDataTypeStr=boolean
  Relational Operator : RelationalOperator  OutDataTypeStr=boolean  RndMeth=Nearest
  Relational Operator1 : RelationalOperator  Operator=<=  OutDataTypeStr=boolean  RndMeth=Nearest
  SampleHold : Subsystem
  Ready : Outport
  wires:
  Canal1/1 -> Relational Operator1/1, Relational Operator/1
  HighThreshold/1 -> Relational Operator/2
  isReady/1 -> Logical Operator1/1, SampleHold/2(In2)
  Enable/1 -> Logical Operator2/2
  LowThreshold/1 -> Relational Operator1/2
  Logical Operator/1 -> SampleHold/1(Trigger)
  Logical Operator1/1 -> Logical Operator/2
  Logical Operator2/1 -> Ready/1
  Logical Operator4/1 -> Logical Operator/1
  Relational Operator/1 -> Logical Operator4/2
  Relational Operator1/1 -> Logical Operator4/1
  SampleHold/1(" ") -> Logical Operator2/1

== system gm_Test_DOA/Maximum Hydro 1/SampleHold ==
  Trigger : Inport  OutDataTypeStr=boolean  PortDimensions=1  SampleTime=1e-07
  In2 : Inport  Port=2  OutDataTypeStr=fixdt(1, 18, 0)  PortDimensions=1  SampleTime=1e-07
  Sample and Hold : Subsystem  mask(Sample and Hold){trig=Falling edge, initCond=double(0), latchinput=off}
      mask prompts: trig "Trigger type:"; initCond "Initial condition:"; latchinput "Latch (buffer) input"
      mask help: Sample and hold the input signal. If Latch (buffer) input is selected, then this block produces the value of the input from the previous time step.
      mask init:
      | switch trig
      | case 1, s='rising';
      | case 2, s='falling';
      | case 3, s='either';
      | end
      | set_param([gcb '/Trigger'],'triggertype',s);
      | if (latchinput == 1)
      | 	set_param([gcb '/In'],'latchinput','on');
      | else
      | 	set_param([gcb '/In'],'latchinput','off');
      | end
      mask Help: eval('blocksethelp');
      mask TypeOptions trig: Rising edge | Falling edge | Either edge
      mask Display: disp('S/H')
  " " : Outport
  wires:
  Trigger/1 -> Sample and Hold/Trigger
  In2/1 -> Sample and Hold/1(In)
  Sample and Hold/1(" ") -> " "/1

== system gm_Test_DOA/Maximum Hydro 1/SampleHold5 ==
  Trigger : Inport  OutDataTypeStr=boolean  PortDimensions=1  SampleTime=1e-07
  In2 : Inport  Port=2  OutDataTypeStr=fixdt(1, 20, 17)  PortDimensions=1  SampleTime=1e-07
  Sample and Hold : Subsystem  mask(Sample and Hold){trig=Falling edge, initCond=double(0), latchinput=off}
      mask prompts: trig "Trigger type:"; initCond "Initial condition:"; latchinput "Latch (buffer) input"
      mask help: Sample and hold the input signal. If Latch (buffer) input is selected, then this block produces the value of the input from the previous time step.
      mask init: same as gm_Test_DOA/Maximum Hydro 1/SampleHold/Sample and Hold
      mask Help: eval('blocksethelp');
      mask TypeOptions trig: Rising edge | Falling edge | Either edge
      mask Display: disp('S/H')
  " " : Outport
  wires:
  Trigger/1 -> Sample and Hold/Trigger
  In2/1 -> Sample and Hold/1(In)
  Sample and Hold/1(" ") -> " "/1

== system gm_Test_DOA/Maximum Hydro 1/SampleHold6 ==
  Trigger : Inport  OutDataTypeStr=boolean  PortDimensions=1  SampleTime=1e-07
  In2 : Inport  Port=2  OutDataTypeStr=fixdt(1, 20, 17)  PortDimensions=1  SampleTime=1e-07
  Sample and Hold : Subsystem  mask(Sample and Hold){trig=Falling edge, initCond=double(0), latchinput=off}
      mask prompts: trig "Trigger type:"; initCond "Initial condition:"; latchinput "Latch (buffer) input"
      mask help: Sample and hold the input signal. If Latch (buffer) input is selected, then this block produces the value of the input from the previous time step.
      mask init: same as gm_Test_DOA/Maximum Hydro 1/SampleHold/Sample and Hold
      mask Help: eval('blocksethelp');
      mask TypeOptions trig: Rising edge | Falling edge | Either edge
      mask Display: disp('S/H')
  " " : Outport
  wires:
  Sample and Hold/1(" ") -> " "/1
  In2/1 -> Sample and Hold/1(In)
  Trigger/1 -> Sample and Hold/Trigger

== system gm_Test_DOA/Maximum Hydro 1/Subsystem ==
  Enable/Reset : Inport  OutDataTypeStr=boolean  PortDimensions=1  SampleTime=1e-07
  Add : Sum
  Data Type Conversion1 : DataTypeConversion  OutDataTypeStr=uint16  RndMeth=Nearest
  Delay : Delay  DelayLength=1  InitialCondition=0  UseCircularBuffer=on
  Product2 : Product
  Count : Outport  VectorParamsAs1DForOutWhenUnconnected=off
  wires:
  Enable/Reset/1 -> Product2/1, Add/1
  Add/1 -> Product2/2
  Data Type Conversion1/1 -> Add/2
  Delay/1 -> Data Type Conversion1/1, Count/1
  Product2/1 -> Delay/1

== system gm_Test_DOA/Maximum Hydro 2/SampleHold ==
  Trigger : Inport  OutDataTypeStr=boolean  PortDimensions=1  SampleTime=1e-07
  In2 : Inport  Port=2  OutDataTypeStr=fixdt(1, 18, 0)  PortDimensions=1  SampleTime=1e-07
  Sample and Hold : Subsystem  mask(Sample and Hold){trig=Falling edge, initCond=double(0), latchinput=off}
      mask prompts: trig "Trigger type:"; initCond "Initial condition:"; latchinput "Latch (buffer) input"
      mask help: Sample and hold the input signal. If Latch (buffer) input is selected, then this block produces the value of the input from the previous time step.
      mask init: same as gm_Test_DOA/Maximum Hydro 1/SampleHold/Sample and Hold
      mask Help: eval('blocksethelp');
      mask TypeOptions trig: Rising edge | Falling edge | Either edge
      mask Display: disp('S/H')
  " " : Outport
  wires:
  Sample and Hold/1(" ") -> " "/1
  In2/1 -> Sample and Hold/1(In)
  Trigger/1 -> Sample and Hold/Trigger

== system gm_Test_DOA/Maximum Hydro 2/SampleHold5 ==
  Trigger : Inport  OutDataTypeStr=boolean  PortDimensions=1  SampleTime=1e-07
  In2 : Inport  Port=2  OutDataTypeStr=fixdt(1, 20, 17)  PortDimensions=1  SampleTime=1e-07
  Sample and Hold : Subsystem  mask(Sample and Hold){trig=Falling edge, initCond=double(0), latchinput=off}
      mask prompts: trig "Trigger type:"; initCond "Initial condition:"; latchinput "Latch (buffer) input"
      mask help: Sample and hold the input signal. If Latch (buffer) input is selected, then this block produces the value of the input from the previous time step.
      mask init: same as gm_Test_DOA/Maximum Hydro 1/SampleHold/Sample and Hold
      mask Help: eval('blocksethelp');
      mask TypeOptions trig: Rising edge | Falling edge | Either edge
      mask Display: disp('S/H')
  " " : Outport
  wires:
  Sample and Hold/1(" ") -> " "/1
  In2/1 -> Sample and Hold/1(In)
  Trigger/1 -> Sample and Hold/Trigger

== system gm_Test_DOA/Maximum Hydro 2/SampleHold6 ==
  Trigger : Inport  OutDataTypeStr=boolean  PortDimensions=1  SampleTime=1e-07
  In2 : Inport  Port=2  OutDataTypeStr=fixdt(1, 20, 17)  PortDimensions=1  SampleTime=1e-07
  Sample and Hold : Subsystem  mask(Sample and Hold){trig=Falling edge, initCond=double(0), latchinput=off}
      mask prompts: trig "Trigger type:"; initCond "Initial condition:"; latchinput "Latch (buffer) input"
      mask help: Sample and hold the input signal. If Latch (buffer) input is selected, then this block produces the value of the input from the previous time step.
      mask init: same as gm_Test_DOA/Maximum Hydro 1/SampleHold/Sample and Hold
      mask Help: eval('blocksethelp');
      mask TypeOptions trig: Rising edge | Falling edge | Either edge
      mask Display: disp('S/H')
  " " : Outport
  wires:
  Sample and Hold/1(" ") -> " "/1
  In2/1 -> Sample and Hold/1(In)
  Trigger/1 -> Sample and Hold/Trigger

== system gm_Test_DOA/Maximum Hydro 2/Subsystem ==
  Enable/Reset : Inport  OutDataTypeStr=boolean  PortDimensions=1  SampleTime=1e-07
  Add : Sum
  Data Type Conversion1 : DataTypeConversion  OutDataTypeStr=uint16  RndMeth=Nearest
  Delay : Delay  DelayLength=1  InitialCondition=0  UseCircularBuffer=on
  Product2 : Product
  Count : Outport  VectorParamsAs1DForOutWhenUnconnected=off
  wires:
  Enable/Reset/1 -> Product2/1, Add/1
  Add/1 -> Product2/2
  Data Type Conversion1/1 -> Add/2
  Delay/1 -> Data Type Conversion1/1, Count/1
  Product2/1 -> Delay/1

== system gm_Test_DOA/Maximum Hydro 3/SampleHold ==
  Trigger : Inport  OutDataTypeStr=boolean  PortDimensions=1  SampleTime=1e-07
  In2 : Inport  Port=2  OutDataTypeStr=fixdt(1, 18, 0)  PortDimensions=1  SampleTime=1e-07
  Sample and Hold : Subsystem  mask(Sample and Hold){trig=Falling edge, initCond=double(0), latchinput=off}
      mask prompts: trig "Trigger type:"; initCond "Initial condition:"; latchinput "Latch (buffer) input"
      mask help: Sample and hold the input signal. If Latch (buffer) input is selected, then this block produces the value of the input from the previous time step.
      mask init: same as gm_Test_DOA/Maximum Hydro 1/SampleHold/Sample and Hold
      mask Help: eval('blocksethelp');
      mask TypeOptions trig: Rising edge | Falling edge | Either edge
      mask Display: disp('S/H')
  " " : Outport
  wires:
  Sample and Hold/1(" ") -> " "/1
  In2/1 -> Sample and Hold/1(In)
  Trigger/1 -> Sample and Hold/Trigger

== system gm_Test_DOA/Maximum Hydro 3/SampleHold5 ==
  Trigger : Inport  OutDataTypeStr=boolean  PortDimensions=1  SampleTime=1e-07
  In2 : Inport  Port=2  OutDataTypeStr=fixdt(1, 20, 17)  PortDimensions=1  SampleTime=1e-07
  Sample and Hold : Subsystem  mask(Sample and Hold){trig=Falling edge, initCond=double(0), latchinput=off}
      mask prompts: trig "Trigger type:"; initCond "Initial condition:"; latchinput "Latch (buffer) input"
      mask help: Sample and hold the input signal. If Latch (buffer) input is selected, then this block produces the value of the input from the previous time step.
      mask init: same as gm_Test_DOA/Maximum Hydro 1/SampleHold/Sample and Hold
      mask Help: eval('blocksethelp');
      mask TypeOptions trig: Rising edge | Falling edge | Either edge
      mask Display: disp('S/H')
  " " : Outport
  wires:
  Sample and Hold/1(" ") -> " "/1
  In2/1 -> Sample and Hold/1(In)
  Trigger/1 -> Sample and Hold/Trigger

== system gm_Test_DOA/Maximum Hydro 3/SampleHold6 ==
  Trigger : Inport  OutDataTypeStr=boolean  PortDimensions=1  SampleTime=1e-07
  In2 : Inport  Port=2  OutDataTypeStr=fixdt(1, 20, 17)  PortDimensions=1  SampleTime=1e-07
  Sample and Hold : Subsystem  mask(Sample and Hold){trig=Falling edge, initCond=double(0), latchinput=off}
      mask prompts: trig "Trigger type:"; initCond "Initial condition:"; latchinput "Latch (buffer) input"
      mask help: Sample and hold the input signal. If Latch (buffer) input is selected, then this block produces the value of the input from the previous time step.
      mask init: same as gm_Test_DOA/Maximum Hydro 1/SampleHold/Sample and Hold
      mask Help: eval('blocksethelp');
      mask TypeOptions trig: Rising edge | Falling edge | Either edge
      mask Display: disp('S/H')
  " " : Outport
  wires:
  Sample and Hold/1(" ") -> " "/1
  In2/1 -> Sample and Hold/1(In)
  Trigger/1 -> Sample and Hold/Trigger

== system gm_Test_DOA/Maximum Hydro 3/Subsystem ==
  Enable/Reset : Inport  OutDataTypeStr=boolean  PortDimensions=1  SampleTime=1e-07
  Add : Sum
  Data Type Conversion1 : DataTypeConversion  OutDataTypeStr=uint16  RndMeth=Nearest
  Delay : Delay  DelayLength=1  InitialCondition=0  UseCircularBuffer=on
  Product2 : Product
  Count : Outport  VectorParamsAs1DForOutWhenUnconnected=off
  wires:
  Enable/Reset/1 -> Product2/1, Add/1
  Add/1 -> Product2/2
  Data Type Conversion1/1 -> Add/2
  Delay/1 -> Data Type Conversion1/1, Count/1
  Product2/1 -> Delay/1

== system gm_Test_DOA/Maximum Hydro Ref/SampleHold ==
  Trigger : Inport  OutDataTypeStr=boolean  PortDimensions=1  SampleTime=1e-07
  In2 : Inport  Port=2  OutDataTypeStr=fixdt(1, 18, 0)  PortDimensions=1  SampleTime=1e-07
  Sample and Hold : Subsystem  mask(Sample and Hold){trig=Falling edge, initCond=double(0), latchinput=off}
      mask prompts: trig "Trigger type:"; initCond "Initial condition:"; latchinput "Latch (buffer) input"
      mask help: Sample and hold the input signal. If Latch (buffer) input is selected, then this block produces the value of the input from the previous time step.
      mask init: same as gm_Test_DOA/Maximum Hydro 1/SampleHold/Sample and Hold
      mask Help: eval('blocksethelp');
      mask TypeOptions trig: Rising edge | Falling edge | Either edge
      mask Display: disp('S/H')
  " " : Outport
  wires:
  Sample and Hold/1(" ") -> " "/1
  In2/1 -> Sample and Hold/1(In)
  Trigger/1 -> Sample and Hold/Trigger

== system gm_Test_DOA/Maximum Hydro Ref/SampleHold2 ==
  Trigger : Inport  OutDataTypeStr=boolean  PortDimensions=1  SampleTime=1e-07
  In2 : Inport  Port=2  OutDataTypeStr=fixdt(1, 18, 0)  PortDimensions=1  SampleTime=1e-07
  Sample and Hold : Subsystem  mask(Sample and Hold){trig=Falling edge, initCond=double(0), latchinput=off}
      mask prompts: trig "Trigger type:"; initCond "Initial condition:"; latchinput "Latch (buffer) input"
      mask help: Sample and hold the input signal. If Latch (buffer) input is selected, then this block produces the value of the input from the previous time step.
      mask init: same as gm_Test_DOA/Maximum Hydro 1/SampleHold/Sample and Hold
      mask Help: eval('blocksethelp');
      mask TypeOptions trig: Rising edge | Falling edge | Either edge
      mask Display: disp('S/H')
  " " : Outport
  wires:
  Sample and Hold/1(" ") -> " "/1
  In2/1 -> Sample and Hold/1(In)
  Trigger/1 -> Sample and Hold/Trigger

== system gm_Test_DOA/Maximum Hydro Ref/SampleHold3 ==
  Trigger : Inport  OutDataTypeStr=boolean  PortDimensions=1  SampleTime=1e-07
  In2 : Inport  Port=2  OutDataTypeStr=fixdt(0, 17, 0)  PortDimensions=1  SampleTime=1e-07
  Sample and Hold : Subsystem  mask(Sample and Hold){trig=Falling edge, initCond=double(0), latchinput=off}
      mask prompts: trig "Trigger type:"; initCond "Initial condition:"; latchinput "Latch (buffer) input"
      mask help: Sample and hold the input signal. If Latch (buffer) input is selected, then this block produces the value of the input from the previous time step.
      mask init: same as gm_Test_DOA/Maximum Hydro 1/SampleHold/Sample and Hold
      mask Help: eval('blocksethelp');
      mask TypeOptions trig: Rising edge | Falling edge | Either edge
      mask Display: disp('S/H')
  " " : Outport
  wires:
  Trigger/1 -> Sample and Hold/Trigger
  In2/1 -> Sample and Hold/1(In)
  Sample and Hold/1(" ") -> " "/1

== system gm_Test_DOA/Maximum Hydro Ref/SampleHold4 ==
  Trigger : Inport  OutDataTypeStr=boolean  PortDimensions=1  SampleTime=1e-07
  In2 : Inport  Port=2  OutDataTypeStr=fixdt(0, 17, 0)  PortDimensions=1  SampleTime=1e-07
  Sample and Hold : Subsystem  mask(Sample and Hold){trig=Falling edge, initCond=double(0), latchinput=off}
      mask prompts: trig "Trigger type:"; initCond "Initial condition:"; latchinput "Latch (buffer) input"
      mask help: Sample and hold the input signal. If Latch (buffer) input is selected, then this block produces the value of the input from the previous time step.
      mask init: same as gm_Test_DOA/Maximum Hydro 1/SampleHold/Sample and Hold
      mask Help: eval('blocksethelp');
      mask TypeOptions trig: Rising edge | Falling edge | Either edge
      mask Display: disp('S/H')
  " " : Outport
  wires:
  Sample and Hold/1(" ") -> " "/1
  In2/1 -> Sample and Hold/1(In)
  Trigger/1 -> Sample and Hold/Trigger

== system gm_Test_DOA/Maximum Hydro Ref/SampleHold5 ==
  Trigger : Inport  OutDataTypeStr=boolean  PortDimensions=1  SampleTime=1e-07
  In2 : Inport  Port=2  OutDataTypeStr=fixdt(1, 20, 17)  PortDimensions=1  SampleTime=1e-07
  Sample and Hold : Subsystem  mask(Sample and Hold){trig=Falling edge, initCond=double(0), latchinput=off}
      mask prompts: trig "Trigger type:"; initCond "Initial condition:"; latchinput "Latch (buffer) input"
      mask help: Sample and hold the input signal. If Latch (buffer) input is selected, then this block produces the value of the input from the previous time step.
      mask init: same as gm_Test_DOA/Maximum Hydro 1/SampleHold/Sample and Hold
      mask Help: eval('blocksethelp');
      mask TypeOptions trig: Rising edge | Falling edge | Either edge
      mask Display: disp('S/H')
  " " : Outport
  wires:
  Sample and Hold/1(" ") -> " "/1
  In2/1 -> Sample and Hold/1(In)
  Trigger/1 -> Sample and Hold/Trigger

== system gm_Test_DOA/Maximum Hydro Ref/SampleHold6 ==
  Trigger : Inport  OutDataTypeStr=boolean  PortDimensions=1  SampleTime=1e-07
  In2 : Inport  Port=2  OutDataTypeStr=fixdt(1, 20, 17)  PortDimensions=1  SampleTime=1e-07
  Sample and Hold : Subsystem  mask(Sample and Hold){trig=Falling edge, initCond=double(0), latchinput=off}
      mask prompts: trig "Trigger type:"; initCond "Initial condition:"; latchinput "Latch (buffer) input"
      mask help: Sample and hold the input signal. If Latch (buffer) input is selected, then this block produces the value of the input from the previous time step.
      mask init: same as gm_Test_DOA/Maximum Hydro 1/SampleHold/Sample and Hold
      mask Help: eval('blocksethelp');
      mask TypeOptions trig: Rising edge | Falling edge | Either edge
      mask Display: disp('S/H')
  " " : Outport
  wires:
  Sample and Hold/1(" ") -> " "/1
  In2/1 -> Sample and Hold/1(In)
  Trigger/1 -> Sample and Hold/Trigger
